simulink model "e8_PMSM_SprayMultiNozzle_ROM"  (R2021b)
settings: Solver=VariableStepAuto  StartTime=0.0  StopTime=1000  RelTol=1e-3  AbsTol=1e-3
model workspace (MAT data in the model file):
  AdjacencyMat = [0 0 0 0 0 0 0 0 0 0 0 0 ... (12996 elements, 114x114)]
  Banding_Loss_Mat = [0 0 0 0 0 0 0 0 0 0 0 0 ... (2340 elements, 39x60)]
  CapMat = [1e+20 2196.70091586 387.653102799 193.8265514 1962.34710525 387.653102799 193.8265514 1962.34710525 1266.59353814 268.053957132 416.539515956 175.715078 ... (114 elements, 114x1)]
  CoolantArrayIdxs = [21; 29; 78; 100; 30; 31; 32; 33]
  Friction_Loss_Mat = [0 0 0 0 0 0 0 0 0 0 0 0 ... (2340 elements, 39x60)]
  InletCoolIdxs = [30  31  32  33; 29  29  29  29; 30  31  32  33]
  Iron_Loss_Rotor_Back_Iron_Mat = [0.0117705351991 0.0200087653806 0.0246811430764 0.0256578010281 0.0240025552689 0.0207013457731 0.0167627779958 0.013305715839 0.0115602539828 0.0121149481083 0.0143511671725 0.0171856755847 ... (2340 elements, 39x60)]
  Iron_Loss_Rotor_Pole_Mat = [1.45649756865 1.45241481649 1.42884898554 1.39022048903 1.34148134724 1.28634015611 1.22776297278 1.16827194649 1.11002512364 1.05393003616 0.999091137463 0.943664155592 ... (2340 elements, 39x60)]
  Iron_Loss_Rotor_Tooth_Mat = [0 0 0 0 0 0 0 0 0 0 0 0 ... (2340 elements, 39x60)]
  Iron_Loss_Stator_Back_Iron_Mat = [38.5419456951 37.7562377622 36.7626331345 35.6659256425 34.5041164064 33.3097183676 32.1148301022 30.9550268851 29.8690226279 28.862614511 27.8706329494 26.7877765024 ... (2340 elements, 39x60)]
  Iron_Loss_Stator_Tooth_Mat = [42.0610884508 41.0367236596 40.1636589805 39.4141834911 38.6901612332 37.9457147976 37.1698474109 36.3762859147 35.5917582202 34.8149830437 33.9858111542 33.0265171037 ... (2340 elements, 39x60)]
  LossDistrForEachType = [0 0 0 0 0 0 0 0 0 0 0 0 ... (2736 elements, 24x114)]
  Magnet_Loss_Mat = [0.0995193918038 0.0927324879203 0.0867464499603 0.0817901209144 0.0773904805464 0.0731587227427 0.068708638331 0.0635818407139 0.057217354686 0.0494585613633 0.0409403305493 0.0325683424692 ... (2340 elements, 39x60)]
  OutletCoolIdxs = [30  31  32  33; 100  100  100  100; 30  31  32  33]
  RotorCopperTempCoefResistivity = 0.00393
  Rotor_Cage_Loss_Mat = [0 0 0 0 0 0 0 0 0 0 0 0 ... (2340 elements, 39x60)]
  ShaftTorqueVec = [-286.936099977 -271.951133863 -256.966167748 -241.981201634 -226.99623552 -212.011269406 -197.026303292 -182.041337178 -167.056371063 -152.071404949 -137.086438835 -122.101472721 ... (39 elements, 1x39)]
  Sleeve_Loss_Mat = [0 0 0 0 0 0 0 0 0 0 0 0 ... (2340 elements, 39x60)]
  SpeedVec = [500 661.016949153 822.033898305 983.050847458 1144.06779661 1305.08474576 1466.10169492 1627.11864407 1788.13559322 1949.15254237 2110.16949153 2271.18644068 ... (60 elements, 1x60)]
  StateSpaceND : object (value not decoded)
  StatorCopperTempCoefResistivity = 0.00393
  Stator_Copper_Loss_AC_Mat = [0 0 0 0 0 0 0 0 0 0 0 0 ... (2340 elements, 39x60)]
  Stator_Copper_Loss_Mat = [3925.33912093 3500.33132705 3080.91358293 2704.55804144 2364.73307434 2056.62848353 1776.61435032 1521.89015388 1290.25886694 1079.99319182 889.737399072 718.403752767 ... (2340 elements, 39x60)]
  Stray_Load_Loss_Mat = [0 0 0 0 0 0 0 0 0 0 0 0 ... (2340 elements, 39x60)]
  Stray_Loss_Stator_Iron_Proportion = 0.95
  TnodesInit = [25 25 25 25 25 25 25 25 25 25 25 25 ... (114 elements, 114x1)]
  TrefRotor = 20
  TrefStator = 20
  Windage_Loss_Mat = [0 0 0 0 0 0 0 0 0 0 0 0 ... (2340 elements, 39x60)]
libraries: mcadROM_lib x4
(part 2 of 2)

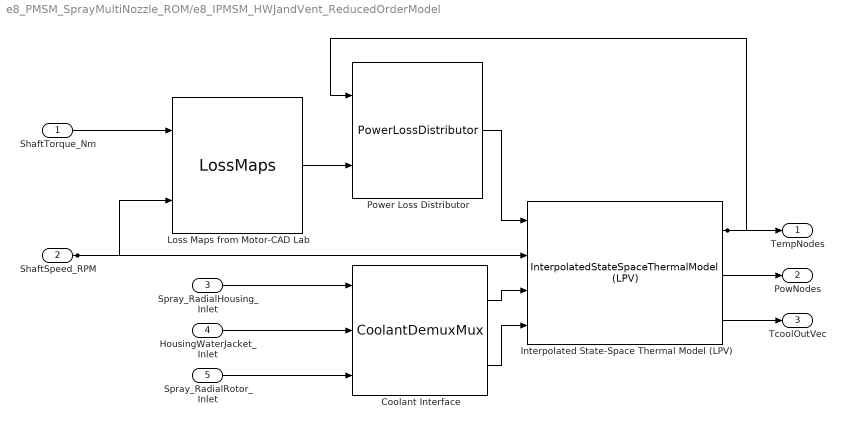
== system e8_PMSM_SprayMultiNozzle_ROM/e8_IPMSM_HWJandVent_ReducedOrderModel ==
  ShaftTorque_Nm : Inport
  ShaftSpeed_RPM : Inport  Port=2
  Spray_RadialHousing_Inlet : Inport  Port=3
  HousingWaterJacket_Inlet : Inport  Port=4
  Spray_RadialRotor_Inlet : Inport  Port=5
  Coolant Interface : mcadROM_lib/CoolantDemuxMux  numCoolSys=3
  Interpolated State-Space Thermal Model (LPV) : mcadROM_lib/InterpolatedStateSpaceThermalModel (LPV)  StateSpaceND=StateSpaceND  CoolAdjMat=AdjacencyMat  CoolantArrayIdxs=CoolantArrayIdxs  InletCoolantIdxs=InletCoolIdxs  OutletCoolantIdxs=OutletCoolIdxs  TnodesInit=TnodesInit
  Loss Maps from Motor-CAD Lab : mcadROM_lib/LossMaps  ShaftTorqueVec=ShaftTorqueVec  SpeedVec=SpeedVec  Stator_Copper_Loss_Mat=Stator_Copper_Loss_Mat  Rotor_Cage_Loss_Mat=Rotor_Cage_Loss_Mat  Iron_Loss_Stator_Back_Iron_Mat=Iron_Loss_Stator_Back_Iron_Mat  Iron_Loss_Stator_Tooth_Mat=Iron_Loss_Stator_Tooth_Mat  Stray_Loss_Stator_Iron_Proportion=Stray_Loss_Stator_Iron_Proportion  Stray_Load_Loss_Mat=Stray_Load_Loss_Mat  Magnet_Loss_Mat=Magnet_Loss_Mat  Iron_Loss_Rotor_Pole_Mat=Iron_Loss_Rotor_Pole_Mat  Iron_Loss_Rotor_Back_Iron_Mat=Iron_Loss_Rotor_Back_Iron_Mat  Iron_Loss_Rotor_Tooth_Mat=Iron_Loss_Rotor_Tooth_Mat  Friction_Loss_Mat=Friction_Loss_Mat  Windage_Loss_Mat=Windage_Loss_Mat  Stator_Copper_Loss_AC_Mat=Stator_Copper_Loss_AC_Mat  Banding_Loss_Mat=Banding_Loss_Mat  Sleeve_Loss_Mat=Sleeve_Loss_Mat
  Power Loss Distributor : mcadROM_lib/PowerLossDistributor  TrefStator=TrefStator  StatorCopperTempCoefResistivity=StatorCopperTempCoefResistivity  TrefRotor=TrefRotor  RotorCopperTempCoefResistivity=RotorCopperTempCoefResistivity  LossDistrForEachType=LossDistrForEachType  CapMat=CapMat  CoolantArrayIdxs=CoolantArrayIdxs
  TempNodes : Outport
  PowNodes : Outport  Port=2
  TcoolOutVec : Outport  Port=3
  wires:
  Interpolated State-Space Thermal Model (LPV)/1 -> Power Loss Distributor/1, TempNodes/1
  Interpolated State-Space Thermal Model (LPV)/3 -> TcoolOutVec/1
  Interpolated State-Space Thermal Model (LPV)/2 -> PowNodes/1
  Coolant Interface/2 -> Interpolated State-Space Thermal Model (LPV)/4
  Coolant Interface/1 -> Interpolated State-Space Thermal Model (LPV)/3
  Spray_RadialRotor_Inlet/1 -> Coolant Interface/3
  HousingWaterJacket_Inlet/1 -> Coolant Interface/2
  ShaftTorque_Nm/1 -> Loss Maps from Motor-CAD Lab/1
  Loss Maps from Motor-CAD Lab/1 -> Power Loss Distributor/2
  Spray_RadialHousing_Inlet/1 -> Coolant Interface/1
  ShaftSpeed_RPM/1 -> Loss Maps from Motor-CAD Lab/2, Interpolated State-Space Thermal Model (LPV)/2
  Power Loss Distributor/1 -> Interpolated State-Space Thermal Model (LPV)/1
